simulink model "clutchmodel_V2"  (R2016a)
settings: Solver=ode45  StartTime=0.0  StopTime=3  RelTol=1e-3
PreLoadFcn:
  | %% parameters of model
  | SlopeGrade = 0   % SlopeGrade deg
  | 
  | %%%%%%%%%%%%%%%%%%%%%%%%%%%%%%%%%%%%%%%%%%%%%%%%%%%%%%%%%%%%%%%%%%% Engine
  | I_e=0.16;   % moment of crank [kgm2]
  | C_e=0.06;   % damping coefficient at the engine [Nm/(rad/s)]
  | 
  | %%%%%%%%%%%%%%%%%%%%%%%%%%%%%%%%%%%%%%%%%%%%%%%%%%%%%%%%%%%%%%%%%%% Clutch
  | mu = 0.4;
  | D = 0.22;       % diameter on clutch friction plate
  | R_c = D/2;
  | 
  | %%%%%%%%%%%%%%%%%%%%%%%%%%%%%%%%%%%%%%%%%%%%%%%%%%%%%%%%%%%%%%%%%%% Transmission
  | i1 = 34.45/10;          % transmission ratio of 1st gear
  | 
  | %%%%%%%%%%%%%%%%%%%%%%%%%%%%%%%%%%%%%%%%%%%%%%%%%%%%%%%%%%%%%%%%%%% Shaft
  | Rfd = 45.33/10;         % Final Driver Ratio
  | C_v = 0.08;             % Nm/(rad/s) damp of driveline
  | 
  | %%%%%%%%%%%%%%%%%%%%%%%%%%%%%%%%%%%%%%%%%%%%%%%%%%%%%%%%%%%%%%%%%%% Tires and Vehicle
  | m = 1500; % kg
  | g = 9.8;
  | mu_r = 0.02;
  | rload0 = 100;      % drag friction at wheels   Nm
  | rload2 = 0.7*1.5/1.6319;  % airodynamic drag CD*A*u^2/1.6319 = 0.7*6/1.6319*u^2 = 2.57*u^2
  | Rw = 0.317; %  wheel radius  m
  | I_v = m*Rw^2/(i1*Rfd)^2;      % value of vehicle inertia (kgm^2)
values from neighbouring files (symbols this model uses):
  K_d = N*hd0    [clutch_v2.m]
  K_d1 = N*hd1    [clutch_v2.m]
undefined symbols (not defined in the file or in its folder): K_p1, K_p2, K_p3, K_x1, K_x2
settings Model: Creator=Administrator  LastModifiedBy=lenovo
settings DataIOCC: LimitDataPoints=on  SaveFormat=Array
settings DebuggingCC: MaxConsecutiveZCsMsg=none
settings HardwareCC: ProdBitPerPointer=32  ProdLargestAtomicFloat=None  ProdIntDivRoundTo=Undefined  ProdEndianess=Unspecified  ProdWordSize=32  ProdHWDeviceType=32-bit Generic
settings ModelReferenceCC: PropagateSignalLabelsOutOfModel=off
settings ConfigComp: CovModelRefEnable=Off  CovSFcnEnable=off

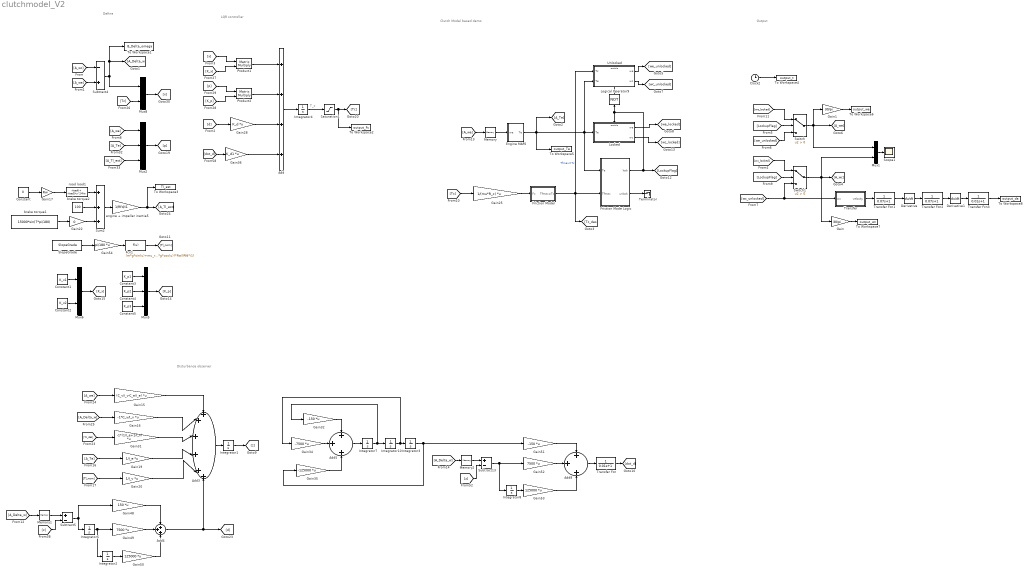
== system clutchmodel_V2 ==
  note: Define
  note: Disturbance observer
  note: T_c
  note: LQR controller
  note: Clutch Model based demo
  note: Output
  Add : Sum  Inputs=++++
  Add3 : Sum  Inputs=++++++
  Add4 : Sum  Inputs=+++
  Add5 : Sum  Inputs=+++
  Add8 : Sum  Inputs=+++
  Clock2 : Clock
  Constant : Constant  Value=0
  Constant1 : Constant  Value=K_x1
  Constant2 : Constant  Value=K_x2
  Constant3 : Constant  Value=K_p1
  Constant4 : Constant  Value=K_p2
  Constant5 : Constant  Value=K_p3
  Derivative : Derivative
  Derivative1 : Derivative
  Engine MAP2 : Subsystem
  Fcn1 : Fcn  Expr=(m*g*sin(u)+mu_r*m*g*cos(u))*Rw/(Rfd*i1)
  Friction Mode Logic : Subsystem
  Friction Model : Subsystem
  Gain : Gain  Gain=30/pi
  Gain1 : Gain  Gain=30/pi
  Gain15 : Gain  Gain=(C_v/I_v-C_e/I_e)  Multiplication=Matrix(K*u)
  Gain16 : Gain  Gain=-1*C_v/I_v  Multiplication=Matrix(K*u)
  Gain17 : Gain  Gain=Rw
  Gain19 : Gain  Gain=1/I_e  Multiplication=Matrix(K*u)
  Gain20 : Gain  Gain=1/I_v  Multiplication=Matrix(K*u)
  Gain22 : Gain  Gain=0
  Gain25 : Gain  Gain=1/(mu*R_c)  Multiplication=Matrix(K*u)
  Gain28 : Gain  Gain=K_d  Multiplication=Matrix(K*u)
  Gain31 : Gain  Gain=-1*(1/I_e+1/I_v)  Multiplication=Matrix(K*u)
  Gain32 : Gain  Gain=-150  Multiplication=Matrix(K*u)
  Gain34 : Gain  Gain=-7500  Multiplication=Matrix(K*u)
  Gain35 : Gain  Gain=-125000  Multiplication=Matrix(K*u)
  Gain36 : Gain  Gain=K_d1  Multiplication=Matrix(K*u)
  Gain48 : Gain  Gain=150  Multiplication=Matrix(K*u)
  Gain49 : Gain  Gain=7500  Multiplication=Matrix(K*u)
  Gain50 : Gain  Gain=125000  Multiplication=Matrix(K*u)
  Gain51 : Gain  Gain=-150  Multiplication=Matrix(K*u)
  Gain52 : Gain  Gain=7500  Multiplication=Matrix(K*u)
  Gain53 : Gain  Gain=125000  Multiplication=Matrix(K*u)
  Gain54 : Gain  Gain=pi/180  Multiplication=Matrix(K*u)
  Integrator1 : Integrator  InitialCondition=83.78
  Integrator{2..3,5,7..8,10} (6 alike) : Integrator
  Integrator4 : Integrator  LimitOutput=on  LowerSaturationLimit=0
  Locked : Subsystem  TreatAsAtomicUnit=on
      mask Display: plot(-1,-6,6,12,[0 3],[3 3],[3 1 1 3], [1 1 5 5],[2 4 4 2],[4 4 2 2],[4 5],[3 3])
  Logical Operator9 : Logic  Operator=NOT  Inputs=1  IconShape=distinctive  OutDataTypeStr=boolean
  Memory : Memory
  Memory1 : Memory
  Memory2 : Memory
  Mux1 : Mux  Inputs=2
  Mux2 : Mux  Inputs=3
  Mux5 : Mux  Inputs=3
  Mux6 : Mux  Inputs=2
  Mux8 : Mux  Inputs=2
  Product1 : Product  Multiplication=Matrix(*)
  Product2 : Product  Multiplication=Matrix(*)
  Saturation1 : Saturate  UpperLimit=188  LowerLimit=0
  Scope1 : Scope
  SlopeGrade : Constant  Value=SlopeGrade
  Subtract13 : Sum  Inputs=+-
  Subtract4 : Sum  Inputs=-+
  Subtract5 : Sum  Inputs=+-
  Sum2 : Sum  Inputs=+++  SaturateOnIntegerOverflow=on  InputSameDT=on  OutDataTypeStr=Inherit: Same as first input
  Switch : Switch  Criteria=u2 > Threshold
  Switch1 : Switch  Criteria=u2 > Threshold
  Terminator : Terminator
  To Workspace1 : ToWorkspace  VariableName=B_Delta_omega  SaveFormat=Structure With Time  SampleTime=-1
  To Workspace2 : ToWorkspace  VariableName=output_Fc  SampleTime=-1
      settings: Save2DSignal=2-D array (concatenate along first dimension)
  To Workspace3 : ToWorkspace  VariableName=Tl_est  SaveFormat=Structure With Time  SampleTime=-1
  To Workspace4 : ToWorkspace  VariableName=output_t  SampleTime=-1
  To Workspace5 : ToWorkspace  VariableName=output_Te  SampleTime=-1
      settings: Save2DSignal=2-D array (concatenate along first dimension)
  To Workspace6 : ToWorkspace  VariableName=output_we  SampleTime=-1
      settings: Save2DSignal=2-D array (concatenate along first dimension)
  To Workspace7 : ToWorkspace  VariableName=output_wc  SampleTime=-1
      settings: Save2DSignal=2-D array (concatenate along first dimension)
  To Workspace8 : ToWorkspace  VariableName=output_da  SampleTime=-1
      settings: Save2DSignal=2-D array (concatenate along first dimension)
  Transfer : Subsystem
  Transfer Fcn : TransferFcn  Denominator=[0.01 1]
  Transfer Fcn1 : TransferFcn  Denominator=[0.07 1]
  Transfer Fcn2 : TransferFcn  Denominator=[0.07 1]
  Transfer Fcn3 : TransferFcn  Denominator=[0.01 1]
  Unlocked : Subsystem  TreatAsAtomicUnit=on
      mask Display: plot(-1,-2,6,8,[0 3],[3 3],[3 1 1 3], [1 1 5 5],[2 4 4 2],[4 4 2 2],[4 5],[3 3])
  brake torque1 : Constant  Value=15000*sin(7*pi/180)
  brake torque2 : Constant  Value=100
  engine + impeller inertia5 : Gain  Gain=1/Rfd/i1  SaturateOnIntegerOverflow=on  OutDataTypeStr=Inherit: Same as input  ParamDataTypeStr=Inherit: Same as input
  road load1 : Fcn  Expr=rload0 + rload2*u^2*Rw
  wires:
  Subtract4/1 -> Mux8/1, To Workspace1/1, [A_Delta_w]
  [Tc] -> Mux8/2
  Mux8/1 -> [x]
  [A_Te] -> Mux2/2
  [A_Tl_est] -> Mux2/3
  Mux2/1 -> [p]
  road load1/1 -> Sum2/1
  brake torque2/1 -> Sum2/2
  Sum2/1 -> engine + impeller inertia5/1
  Constant/1 -> Gain17/1
  Gain17/1 -> road load1/1
  engine + impeller inertia5/1 -> To Workspace3/1, [A_Tl_est]
  brake torque1/1 -> Gain22/1
  Gain22/1 -> Sum2/3
  SlopeGrade/1 -> Gain54/1
  Fcn1/1 -> [Tl_nom]
  Gain54/1 -> Fcn1/1
  [A_we] -> Gain15/1
  [A_Delta_w] -> Gain16/1
  [Tc_des] -> Gain31/1
  [A_Te] -> Gain19/1
  [Tl_nom] -> Gain20/1
  [A_Delta_w] -> Memory1/1
  Add3/1 -> Integrator1/1
  [z] -> Subtract5/2
  Subtract5/1 -> Gain48/1, Integrator5/1
  Gain48/1 -> Add4/1
  Gain49/1 -> Add4/2
  Integrator5/1 -> Integrator2/1, Gain49/1
  Gain31/1 -> Add3/3
  Gain16/1 -> Add3/2
  Gain19/1 -> Add3/4
  Gain15/1 -> Add3/1
  Gain20/1 -> Add3/5
  Integrator1/1 -> [z]
  Add4/1 -> Add3/6, [d]
  Integrator2/1 -> Gain50/1
  Gain50/1 -> Add4/3
  Add5/1 -> Integrator7/1
  Gain34/1 -> Add5/2
  Gain32/1 -> Add5/1
  Gain35/1 -> Add5/3
  Integrator7/1 -> Gain32/1, Integrator10/1
  Gain51/1 -> Add8/1
  Gain52/1 -> Add8/2
  Gain53/1 -> Add8/3
  [A_Delta_w] -> Memory2/1
  [z] -> Subtract13/2
  Subtract13/1 -> Integrator8/1, Gain52/1
  Integrator8/1 -> Gain53/1
  Add8/1 -> Transfer Fcn/1
  Transfer Fcn/1 -> [dot_d]
  [d] -> Gain28/1
  Product1/1 -> Add/1
  Add/1 -> Integrator4/1
  [x] -> Product1/1
  Product2/1 -> Add/2
  Integrator4/1 -> Saturation1/1
  [dot_d] -> Gain36/1
  Logical Operator9/1 -> Unlocked/Enable
  Friction Model/1(Tfmax=Tc) -> [Tc_des], Unlocked/1(Tc), Friction Mode Logic/2(Tfmax)  "Tfmax=Tc"
  Gain25/1 -> Friction Model/1(Fc)
  Friction Mode Logic/1(lock) -> Locked/Enable, Logical Operator9/1, [LockupFlag]
  Friction Mode Logic/2(unlock) -> Terminator/1
  [LockupFlag] -> Switch/2
  [we_unlocked] -> Switch/3
  [we_locked] -> Switch/1
  [LockupFlag] -> Switch1/2
  [wc_locked] -> Switch1/1
  Locked/1(we) -> [we_locked]
  Unlocked/1(we) -> [we_unlocked]
  Unlocked/2(wc) -> [wc_unlocked]
  Gain36/1 -> Add/4
  Gain28/1 -> Add/3
  Locked/2(wc) -> [wc_locked]
  Mux5/1 -> [K_p]
  Constant3/1 -> Mux5/1
  Constant4/1 -> Mux5/2
  Constant5/1 -> Mux5/3
  Mux6/1 -> [K_x]
  Constant1/1 -> Mux6/1
  Constant2/1 -> Mux6/2
  [K_x] -> Product1/2
  [p] -> Product2/1
  [K_p] -> Product2/2
  Derivative/1 -> Transfer Fcn2/1
  Clock2/1 -> To Workspace4/1
  [A_we] -> Memory/1
  Transfer/1(velocity) -> Transfer Fcn1/1
  Transfer Fcn2/1 -> Derivative1/1
  [A_wc] -> Subtract4/1
  [A_we] -> Subtract4/2
  [A_we] -> Mux2/1
  Switch/1 -> Mux1/1, [A_we], Gain1/1
  Switch1/1 -> Mux1/2, Gain/1, [A_wc]
  Gain/1 -> To Workspace7/1
  Gain1/1 -> To Workspace6/1
  Derivative1/1 -> Transfer Fcn3/1
  Transfer Fcn1/1 -> Derivative/1
  Memory/1 -> Engine MAP2/1("we ")
  Mux1/1 -> Scope1/1
  Integrator10/1 -> Integrator3/1, Gain34/1
  Memory1/1 -> Subtract5/1
  Memory2/1 -> Subtract13/1
  [Tc] -> Gain25/1
  Saturation1/1 -> To Workspace2/1, [Tc]
  Integrator3/1 -> Gain35/1, Gain51/1
  Engine MAP2/1(Te) -> [A_Te], Friction Mode Logic/1(Te), Unlocked/2(Te), Locked/1(Te), To Workspace5/1
  [wc_unlocked] -> Transfer/1(wc), Switch1/3
  Transfer Fcn3/1 -> To Workspace8/1

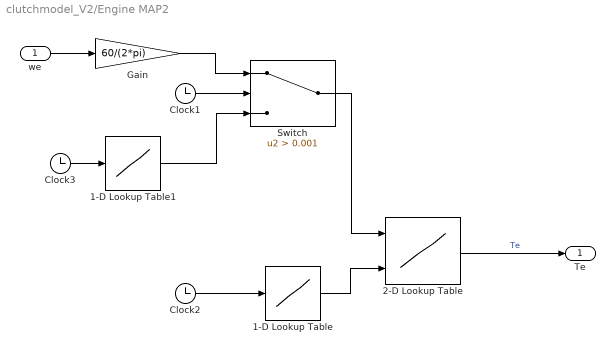
== system clutchmodel_V2/Engine MAP2 ==
  "we " : Inport
  1-D Lookup Table : Lookup_n-D  NumberOfTableDimensions=1  BreakpointsForDimension1=[0 10]  Table=[0.2 0.5]  InternalRulePriority=Speed  RndMeth=Simplest  InputSameDT=on
  1-D Lookup Table1 : Lookup_n-D  NumberOfTableDimensions=1  BreakpointsForDimension1=[0 0.001 ]  Table=[800 800 ]  InternalRulePriority=Speed  RndMeth=Simplest  InputSameDT=on
  2-D Lookup Table : Lookup_n-D  BreakpointsForDimension1=[0;500;1000;2000;3000;4000;5000;6000;6500]  BreakpointsForDimension2=[0 0.2 0.3 0.4 0.6 0.8 1]  Table="[0 0 0 0 0\t0 0;0 85 95 102 103 107.5 110;0 80 100 110 112.5 113.5 115;0 55 105 120 125 127.5 130;0 35\t90 118.5 126 135 137.5;0 24.5 80 122.5 137.5 150 155;0 26 72.5 110 127.5 137.5 140;0 11.5 50 87.5 112.5 125 127.5;0 0 37.5 77.5 110 117.5 117.5]"  InternalRulePriority=Speed  RndMeth=Simplest  InputSameDT=on
  Clock1 : Clock
  Clock2 : Clock
  Clock3 : Clock
  Gain : Gain  Gain=60/(2*pi)
  Switch : Switch  Criteria=u2 > Threshold  Threshold=0.001
  Te : Outport
  wires:
  Switch/1 -> 2-D Lookup Table/1
  1-D Lookup Table/1 -> 2-D Lookup Table/2
  2-D Lookup Table/1 -> Te/1  "Te"
  Clock2/1 -> 1-D Lookup Table/1
  "we "/1 -> Gain/1
  Clock1/1 -> Switch/2
  Gain/1 -> Switch/1
  Clock3/1 -> 1-D Lookup Table1/1
  1-D Lookup Table1/1 -> Switch/3

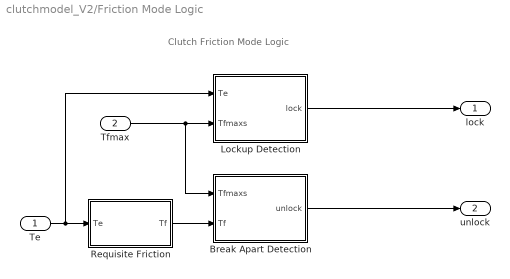
== system clutchmodel_V2/Friction Mode Logic ==
  note: Clutch Friction Mode Logic
  Te : Inport
  Tfmax : Inport  Port=2
  Break Apart Detection : Subsystem
  Lockup Detection : Subsystem
  Requisite Friction : Subsystem
  lock : Outport  InitialOutput=0
  unlock : Outport  Port=2  InitialOutput=0
  wires:
  Lockup Detection/1(lock) -> lock/1
  Break Apart Detection/1(unlock) -> unlock/1
  Requisite Friction/1(Tf) -> Break Apart Detection/2(Tf)
  Tfmax/1 -> Break Apart Detection/1(Tfmaxs), Lockup Detection/2(Tfmaxs)
  Te/1 -> Requisite Friction/1(Te), Lockup Detection/1(Te)

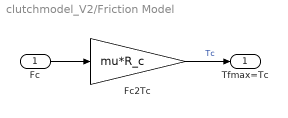
== system clutchmodel_V2/Friction Model ==
  Fc : Inport
  Fc2Tc : Gain  Gain=mu*R_c
  Tfmax=Tc : Outport
  wires:
  Fc/1 -> Fc2Tc/1
  Fc2Tc/1 -> Tfmax=Tc/1  "Tc"

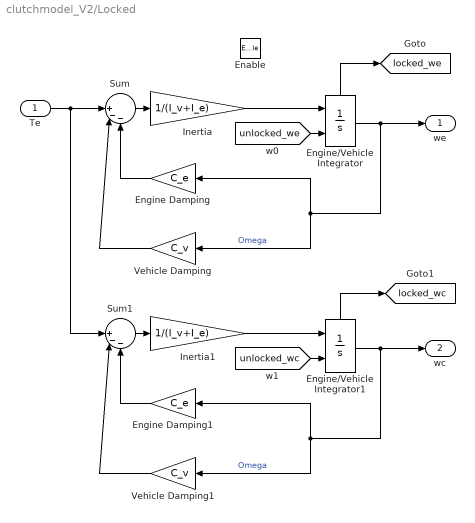
== system clutchmodel_V2/Locked ==
  Te : Inport
  Enable : EnablePort  StatesWhenEnabling=reset
  Engine Damping : Gain  Gain=C_e  SaturateOnIntegerOverflow=on  OutDataTypeStr=Inherit: Same as input  ParamDataTypeStr=Inherit: Same as input
  Engine Damping1 : Gain  Gain=C_e  SaturateOnIntegerOverflow=on  OutDataTypeStr=Inherit: Same as input  ParamDataTypeStr=Inherit: Same as input
  Engine/Vehicle Integrator : Integrator  InitialConditionSource=external  InitialCondition=80  ShowStatePort=on
  Engine/Vehicle Integrator1 : Integrator  InitialConditionSource=external  ShowStatePort=on
  Inertia : Gain  Gain=1/(I_v+I_e)  SaturateOnIntegerOverflow=on  OutDataTypeStr=Inherit: Same as input  ParamDataTypeStr=Inherit: Same as input
  Inertia1 : Gain  Gain=1/(I_v+I_e)  SaturateOnIntegerOverflow=on  OutDataTypeStr=Inherit: Same as input  ParamDataTypeStr=Inherit: Same as input
  Sum : Sum  Inputs=||+--  SaturateOnIntegerOverflow=on  InputSameDT=on  OutDataTypeStr=Inherit: Same as first input
  Sum1 : Sum  Inputs=||+--  SaturateOnIntegerOverflow=on  InputSameDT=on  OutDataTypeStr=Inherit: Same as first input
  Vehicle Damping : Gain  Gain=C_v  SaturateOnIntegerOverflow=on  OutDataTypeStr=Inherit: Same as input  ParamDataTypeStr=Inherit: Same as input
  Vehicle Damping1 : Gain  Gain=C_v  SaturateOnIntegerOverflow=on  OutDataTypeStr=Inherit: Same as input  ParamDataTypeStr=Inherit: Same as input
  we : Outport  InitialOutput=0
  wc : Outport  Port=2  InitialOutput=0
  tag scope: locked_wc=global, locked_we=global
  wires:
  [unlocked_we] -> Engine/Vehicle Integrator/2
  Engine/Vehicle Integrator/State -> [locked_we]
  Sum/1 -> Inertia/1
  Engine/Vehicle Integrator/1 -> we/1, Engine Damping/1, Vehicle Damping/1  "Omega"
  Engine Damping/1 -> Sum/3
  Inertia/1 -> Engine/Vehicle Integrator/1
  Vehicle Damping/1 -> Sum/2
  Sum1/1 -> Inertia1/1
  Te/1 -> Sum1/1, Sum/1
  Engine/Vehicle Integrator1/1 -> wc/1, Engine Damping1/1, Vehicle Damping1/1  "Omega"
  Engine Damping1/1 -> Sum1/3
  Inertia1/1 -> Engine/Vehicle Integrator1/1
  Vehicle Damping1/1 -> Sum1/2
  [unlocked_wc] -> Engine/Vehicle Integrator1/2
  Engine/Vehicle Integrator1/State -> [locked_wc]

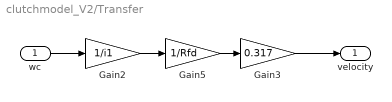
== system clutchmodel_V2/Transfer ==
  wc : Inport
  Gain2 : Gain  Gain=1/i1
  Gain3 : Gain  Gain=0.317
  Gain5 : Gain  Gain=1/Rfd
  velocity : Outport
  wires:
  wc/1 -> Gain2/1
  Gain3/1 -> velocity/1
  Gain5/1 -> Gain3/1
  Gain2/1 -> Gain5/1

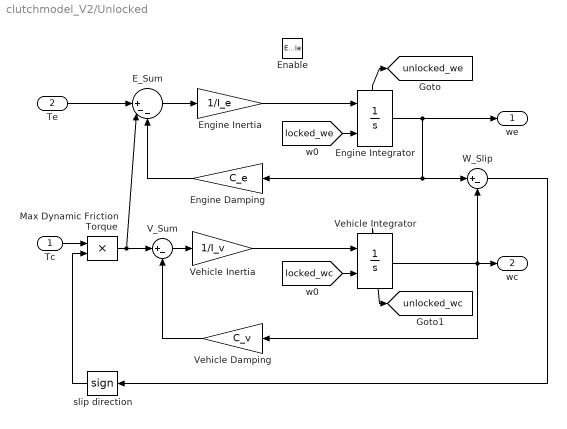
== system clutchmodel_V2/Unlocked ==
  Tc : Inport
  Te : Inport  Port=2
  Enable : EnablePort  StatesWhenEnabling=reset
  E_Sum : Sum  Inputs=||+--  SaturateOnIntegerOverflow=on  InputSameDT=on  OutDataTypeStr=Inherit: Same as first input
  Engine Damping : Gain  Gain=C_e  SaturateOnIntegerOverflow=on  OutDataTypeStr=Inherit: Same as input  ParamDataTypeStr=Inherit: Same as input
  Engine Inertia : Gain  Gain=1/I_e  SaturateOnIntegerOverflow=on  OutDataTypeStr=Inherit: Same as input  ParamDataTypeStr=Inherit: Same as input
  Engine Integrator : Integrator  ExternalReset=rising  InitialCondition=80  ShowStatePort=on
  Max Dynamic Friction Torque : Product  SaturateOnIntegerOverflow=on  RndMeth=Zero  InputSameDT=on  OutDataTypeStr=Inherit: Same as first input
  V_Sum : Sum  Inputs=|+-  SaturateOnIntegerOverflow=on  InputSameDT=on  OutDataTypeStr=Inherit: Same as first input
  Vehicle Damping : Gain  Gain=C_v  SaturateOnIntegerOverflow=on  OutDataTypeStr=Inherit: Same as input  ParamDataTypeStr=Inherit: Same as input
  Vehicle Inertia : Gain  Gain=1/I_v  SaturateOnIntegerOverflow=on  OutDataTypeStr=Inherit: Same as input  ParamDataTypeStr=Inherit: Same as input
  Vehicle Integrator : Integrator  InitialConditionSource=external  ShowStatePort=on
  W_Slip : Sum  Inputs=|+-  SaturateOnIntegerOverflow=on  InputSameDT=on  OutDataTypeStr=Inherit: Same as first input
  slip direction : Signum
  we : Outport  InitialOutput=0
  wc : Outport  Port=2  InitialOutput=0
  tag scope: unlocked_wc=global, unlocked_we=global
  wires:
  V_Sum/1 -> Vehicle Inertia/1
  Vehicle Damping/1 -> V_Sum/2
  Max Dynamic Friction Torque/1 -> V_Sum/1, E_Sum/2
  Tc/1 -> Max Dynamic Friction Torque/1
  slip direction/1 -> Max Dynamic Friction Torque/2
  W_Slip/1 -> slip direction/1
  Engine Integrator/State -> [unlocked_we]
  Engine Inertia/1 -> Engine Integrator/1
  E_Sum/1 -> Engine Inertia/1
  Engine Damping/1 -> E_Sum/3
  Engine Integrator/1 -> we/1, Engine Damping/1, W_Slip/1
  [locked_we] -> Engine Integrator/2
  Te/1 -> E_Sum/1
  Vehicle Integrator/State -> [unlocked_wc]
  [locked_wc] -> Vehicle Integrator/2
  Vehicle Inertia/1 -> Vehicle Integrator/1
  Vehicle Integrator/1 -> wc/1, W_Slip/2, Vehicle Damping/1

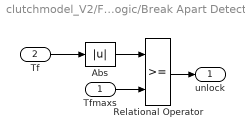
== system clutchmodel_V2/Friction Mode Logic/Break Apart Detection ==
  Tfmaxs : Inport
  Tf : Inport  Port=2
  Abs : Abs  SaturateOnIntegerOverflow=on
  Relational Operator : RelationalOperator  OutDataTypeStr=boolean  InputSameDT=on
  unlock : Outport  InitialOutput=0
  wires:
  Tfmaxs/1 -> Relational Operator/2
  Abs/1 -> Relational Operator/1
  Relational Operator/1 -> unlock/1
  Tf/1 -> Abs/1

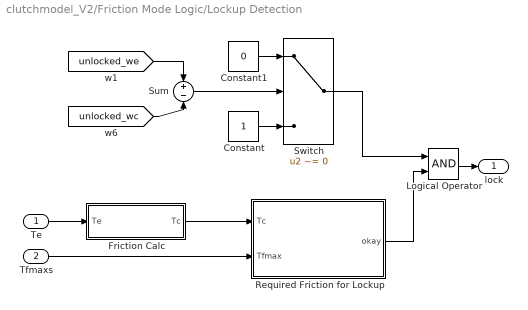
== system clutchmodel_V2/Friction Mode Logic/Lockup Detection ==
  Te : Inport
  Tfmaxs : Inport  Port=2
  Constant : Constant
  Constant1 : Constant  Value=0
  Friction Calc : Subsystem
  Logical Operator : Logic  AllPortsSameDT=off  OutDataTypeStr=boolean
  Required Friction for Lockup : Subsystem
  Sum : Sum  Inputs=+-  SaturateOnIntegerOverflow=on  InputSameDT=on  OutDataTypeStr=Inherit: Same as first input
  Switch : Switch  Criteria=u2 ~= 0
  lock : Outport  InitialOutput=0
  wires:
  Constant/1 -> Switch/3
  Constant1/1 -> Switch/1
  Te/1 -> Friction Calc/1(Te)
  Sum/1 -> Switch/2
  [unlocked_wc] -> Sum/2
  [unlocked_we] -> Sum/1
  Required Friction for Lockup/1(okay) -> Logical Operator/2
  Logical Operator/1 -> lock/1
  Switch/1 -> Logical Operator/1
  Tfmaxs/1 -> Required Friction for Lockup/2(Tfmax)
  Friction Calc/1(Tc) -> Required Friction for Lockup/1(Tc)

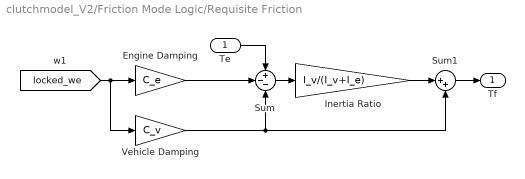
== system clutchmodel_V2/Friction Mode Logic/Requisite Friction ==
  Te : Inport
  Engine Damping : Gain  Gain=C_e  SaturateOnIntegerOverflow=on  OutDataTypeStr=Inherit: Same as input  ParamDataTypeStr=Inherit: Same as input
  Inertia Ratio : Gain  Gain=I_v/(I_v+I_e)  SaturateOnIntegerOverflow=on  OutDataTypeStr=Inherit: Same as input  ParamDataTypeStr=Inherit: Same as input
  Sum : Sum  Inputs=+--  SaturateOnIntegerOverflow=on  InputSameDT=on  OutDataTypeStr=Inherit: Same as first input
  Sum1 : Sum  Inputs=|++  SaturateOnIntegerOverflow=on  InputSameDT=on  OutDataTypeStr=Inherit: Same as first input
  Vehicle Damping : Gain  Gain=C_v  SaturateOnIntegerOverflow=on  OutDataTypeStr=Inherit: Same as input  ParamDataTypeStr=Inherit: Same as input
  Tf : Outport  InitialOutput=0
  wires:
  Sum1/1 -> Tf/1
  Inertia Ratio/1 -> Sum1/1
  Te/1 -> Sum/1
  Sum/1 -> Inertia Ratio/1
  Vehicle Damping/1 -> Sum1/2, Sum/3
  Engine Damping/1 -> Sum/2
  [locked_we] -> Engine Damping/1, Vehicle Damping/1

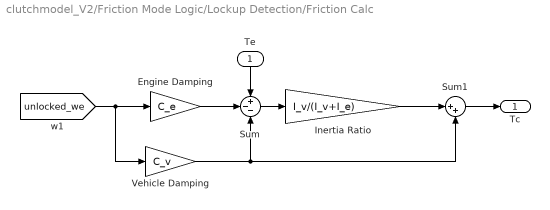
== system clutchmodel_V2/Friction Mode Logic/Lockup Detection/Friction Calc ==
  Te : Inport
  Engine Damping : Gain  Gain=C_e  SaturateOnIntegerOverflow=on  OutDataTypeStr=Inherit: Same as input  ParamDataTypeStr=Inherit: Same as input
  Inertia Ratio : Gain  Gain=I_v/(I_v+I_e)  SaturateOnIntegerOverflow=on  OutDataTypeStr=Inherit: Same as input  ParamDataTypeStr=Inherit: Same as input
  Sum : Sum  Inputs=+--  SaturateOnIntegerOverflow=on  InputSameDT=on  OutDataTypeStr=Inherit: Same as first input
  Sum1 : Sum  Inputs=|++  SaturateOnIntegerOverflow=on  InputSameDT=on  OutDataTypeStr=Inherit: Same as first input
  Vehicle Damping : Gain  Gain=C_v  SaturateOnIntegerOverflow=on  OutDataTypeStr=Inherit: Same as input  ParamDataTypeStr=Inherit: Same as input
  Tc : Outport  InitialOutput=0
  wires:
  Sum1/1 -> Tc/1
  Inertia Ratio/1 -> Sum1/1
  Te/1 -> Sum/1
  Sum/1 -> Inertia Ratio/1
  Engine Damping/1 -> Sum/2
  Vehicle Damping/1 -> Sum/3, Sum1/2
  [unlocked_we] -> Vehicle Damping/1, Engine Damping/1

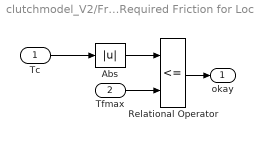
== system clutchmodel_V2/Friction Mode Logic/Lockup Detection/Required Friction for Lockup ==
  Tc : Inport
  Tfmax : Inport  Port=2
  Abs : Abs  SaturateOnIntegerOverflow=on
  Relational Operator : RelationalOperator  Operator=<=  OutDataTypeStr=boolean  InputSameDT=on
  okay : Outport  InitialOutput=0
  wires:
  Tfmax/1 -> Relational Operator/2
  Abs/1 -> Relational Operator/1
  Relational Operator/1 -> okay/1
  Tc/1 -> Abs/1
